simulink model "sustentacao"  (R2025a)
settings: Solver=VariableStepAuto  StartTime=0.0  StopTime=10.0  RelTol=1e-3
libraries: simulink x1
settings Model: Creator=joasb  LastModifiedBy=joasb

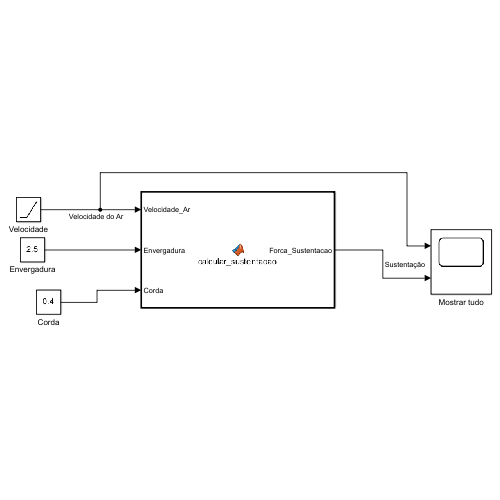
[thumbnail: Simulink's stored preview of the top-level diagram]
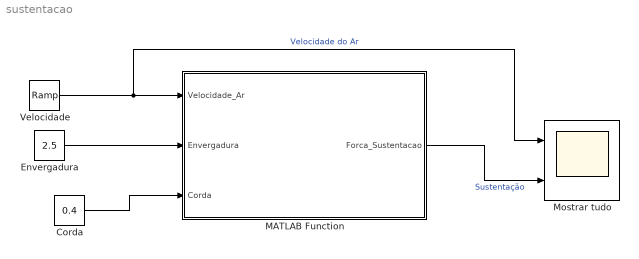
== system sustentacao ==
  Corda : Constant  Value=0.4
  Envergadura : Constant  Value=2.5
  MATLAB Function : MATLAB Function  TreatAsAtomicUnit=on
  Mostrar tudo : Scope  NumInputPorts=2
      settings: ActiveDisplayYMinimum=-9.1874999999999982  ActiveDisplayYMaximum=82.6875
  Velocidade : simulink/Sources/Ramp  slope=1  start=0  InitialOutput=0
  wires:
  Velocidade/1 -> Mostrar tudo/1, MATLAB Function/1(Velocidade_Ar)  "Velocidade do Ar"
  Envergadura/1 -> MATLAB Function/2(Envergadura)
  Corda/1 -> MATLAB Function/3(Corda)
  MATLAB Function/1(Forca_Sustentacao) -> Mostrar tudo/2  "Sustentação"

== matlab function sustentacao/MATLAB Function ==
  data: Velocidade_Ar input; Forca_Sustentacao output; Envergadura input; Corda input
function Forca_Sustentacao = calcular_sustentacao(Velocidade_Ar, Envergadura, Corda)
    
    % Constantes físicas
    rho = 1.225; % Densidade do ar ao nível do mar (kg/m^3)
    Cl = 1.2;    % Coeficiente de sustentação da asa (estimado)
    
    % Cálculo da Área da Asa (S = span * chord, assumindo asa retangular)
    Area_Asa = Envergadura * Corda;
    
    % Calcula a força de sustentação em tempo real
    Forca_Sustentacao = 0.5 * rho * (Velocidade_Ar^2) * Area_Asa * Cl;
    
end
